simulink model "fig3_3_7_text_book"  (R2018b)
settings: Solver=ode4  StartTime=0.0  StopTime=10  FixedStep=.001  RelTol=1e-3
settings Model: Creator=user  LastModifiedBy=user

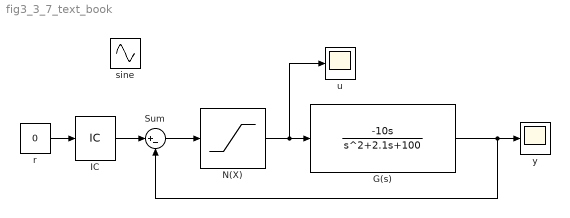
== system fig3_3_7_text_book ==
  G(s) : TransferFcn  Numerator=[-10 0]  Denominator=[1 2.1 100]
  IC : InitialCondition
  N(X) : Saturate  UpperLimit=100  LowerLimit=-100
  Sum : Sum  Inputs=|+-
  r : Constant  Value=0
  "sine " : Sin  Amplitude=3  Frequency=10  SampleTime=0
  u : Scope
  y : Scope
  wires:
  G(s)/1 -> Sum/2, y/1
  N(X)/1 -> u/1, G(s)/1
  Sum/1 -> N(X)/1
  r/1 -> IC/1
  IC/1 -> Sum/1
